simulink model "Assignment2_Simulink"  (R2022b)
settings: Solver=FixedStepAuto  StartTime=0.0  StopTime=20  FixedStep=0.1  RelTol=1e-3
undefined symbols (not defined in the file or in its folder): Ad, Bd, Cd, Dd, k_LQR
libraries: mpclib x6
settings Model: Creator=Alireza  LastModifiedBy=Alireza

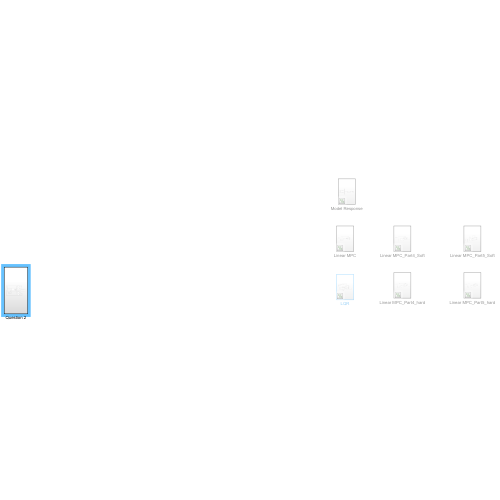
[thumbnail: Simulink's stored preview of the top-level diagram]
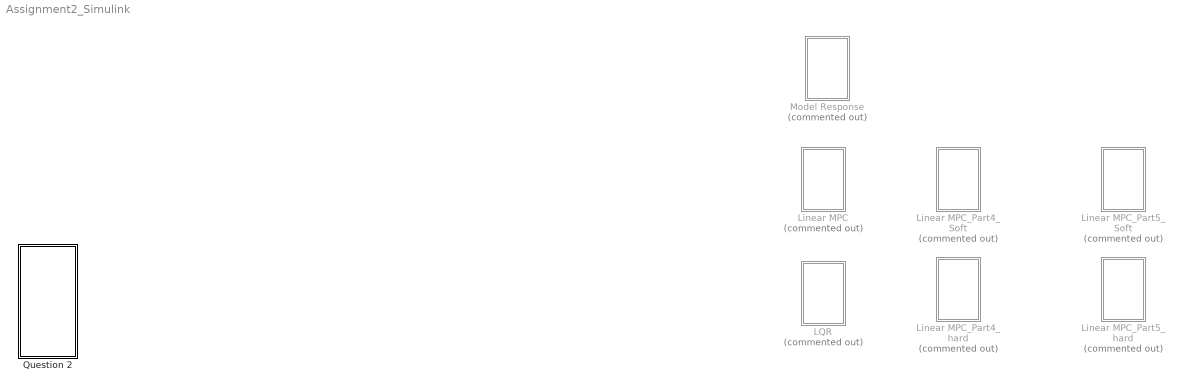
== system Assignment2_Simulink ==
  LQR : Subsystem  Commented=on
  Linear MPC : Subsystem  Commented=on
  Linear MPC_Part4_Soft : Subsystem  Commented=on
  Linear MPC_Part4_hard : Subsystem  Commented=on
  Linear MPC_Part5_Soft : Subsystem  Commented=on
  Linear MPC_Part5_hard : Subsystem  Commented=on
  Model Response : Subsystem  Commented=on
  Question 2 : Subsystem

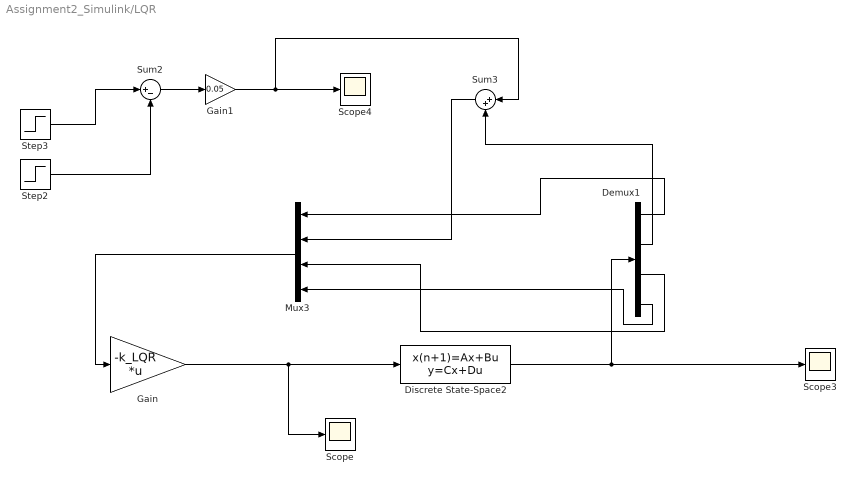
== system Assignment2_Simulink/LQR ==
  Demux1 : Demux
  Discrete State-Space2 : DiscreteStateSpace  A=Ad  B=Bd  C=Cd  D=Dd  InitialCondition=[0,0.1,0,0]  SampleTime=0.1
  Gain : Gain  Gain=-k_LQR  Multiplication=Matrix(K*u)
  Gain1 : Gain  Gain=0.05
  Mux3 : Mux
  Scope : Scope
  Scope3 : Scope
  Scope4 : Scope
  Step2 : Step  Time=5  SampleTime=0
  Step3 : Step  Time=4  SampleTime=0
  Sum2 : Sum  Inputs=|+-
  Sum3 : Sum  Inputs=|++
  wires:
  Demux1/1 -> Mux3/1
  Demux1/3 -> Mux3/3
  Demux1/4 -> Mux3/4
  Sum3/1 -> Mux3/2
  Gain/1 -> Scope/1, Discrete State-Space2/1
  Discrete State-Space2/1 -> Scope3/1, Demux1/1
  Demux1/2 -> Sum3/2
  Step3/1 -> Sum2/1
  Step2/1 -> Sum2/2
  Mux3/1 -> Gain/1
  Sum2/1 -> Gain1/1
  Gain1/1 -> Sum3/1, Scope4/1

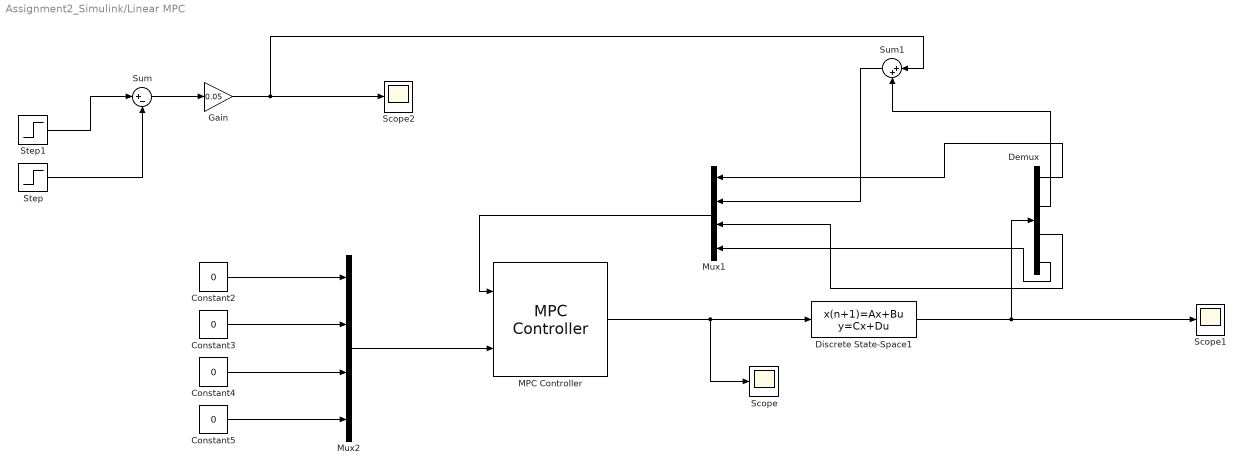
== system Assignment2_Simulink/Linear MPC ==
  Constant{2..5} (4 alike) : Constant  Value=0
  Demux : Demux
  Discrete State-Space1 : DiscreteStateSpace  A=Ad  B=Bd  C=Cd  D=Dd  InitialCondition=[0,0.1,0,0]  SampleTime=0.1
  Gain : Gain  Gain=0.05
  MPC Controller : mpclib/MPC Controller  SCDEnableBlockLinearizationSpecification=on  mpcobj=mpc1  is_multiple=0  enable_value=0  return_u0=off  updateMPCinCallerWorkspace=on  md_inport=off  mv_inport=off  uref_inport=off  return_cost=off  return_mvseq=off  return_qpstatus=off  return_xseq=off  return_state=off  return_ovseq=off  state_inport=off  umin_inport=off  umax_inport=off  ymin_inport=off  ymax_inport=off  cc_inport=off  ywt_inport=off  uwt_inport=off  duwt_inport=off  rhoeps_inport=off  pm_inport=off  MaximumP=10  HorizonChoice=FixedHorizon  n_ts=0.1  n_p=20  n_mv=2  n_md=0  n_ud=0  n_mo=4  n_uo=0  BlockDataType=double  SampleTimeInherited=off  switch_inport=off
  Mux1 : Mux
  Mux2 : Mux
  Scope : Scope
  Scope1 : Scope
  Scope2 : Scope
  Step : Step  Time=5  SampleTime=0
  Step1 : Step  Time=4  SampleTime=0
  Sum : Sum  Inputs=|+-
  Sum1 : Sum  Inputs=|++
  wires:
  Sum1/1 -> Mux1/2
  Step1/1 -> Sum/1
  Discrete State-Space1/1 -> Demux/1, Scope1/1
  Mux2/1 -> MPC Controller/2
  Step/1 -> Sum/2
  Constant3/1 -> Mux2/2
  Mux1/1 -> MPC Controller/1
  Demux/4 -> Mux1/4
  Demux/3 -> Mux1/3
  Constant4/1 -> Mux2/3
  Demux/1 -> Mux1/1
  Constant5/1 -> Mux2/4
  MPC Controller/1 -> Scope/1, Discrete State-Space1/1
  Constant2/1 -> Mux2/1
  Demux/2 -> Sum1/2
  Sum/1 -> Gain/1
  Gain/1 -> Sum1/1, Scope2/1

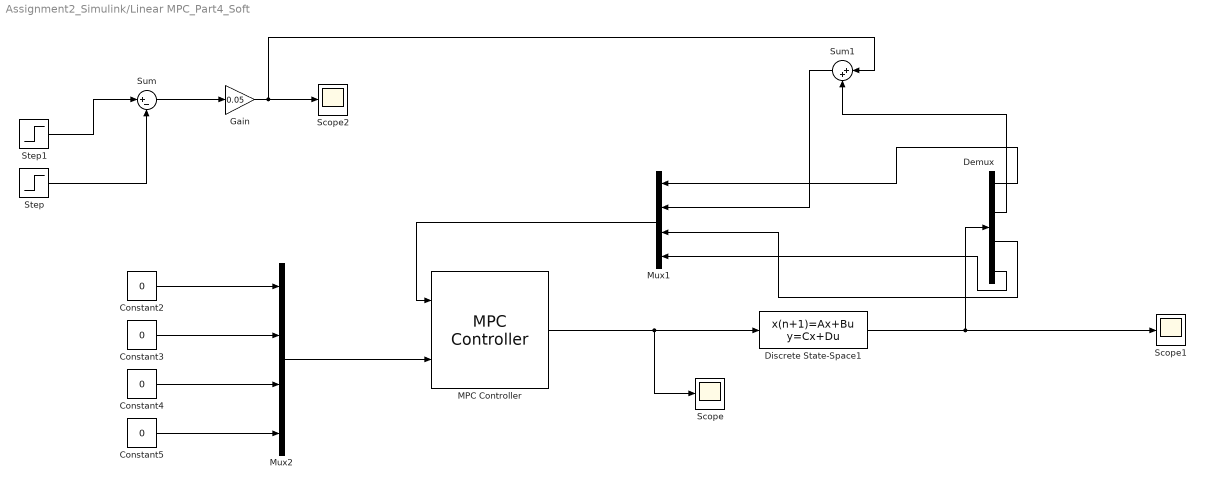
== system Assignment2_Simulink/Linear MPC_Part4_Soft ==
  Constant{2..5} (4 alike) : Constant  Value=0
  Demux : Demux
  Discrete State-Space1 : DiscreteStateSpace  A=Ad  B=Bd  C=Cd  D=Dd  InitialCondition=[0,0.1,0,0]  SampleTime=0.1
  Gain : Gain  Gain=0.05
  MPC Controller : mpclib/MPC Controller  SCDEnableBlockLinearizationSpecification=on  mpcobj=MPC_Part4_Soft  is_multiple=0  enable_value=0  return_u0=off  updateMPCinCallerWorkspace=on  md_inport=off  mv_inport=off  uref_inport=off  return_cost=off  return_mvseq=off  return_qpstatus=off  return_xseq=off  return_state=off  return_ovseq=off  state_inport=off  umin_inport=off  umax_inport=off  ymin_inport=off  ymax_inport=off  cc_inport=off  ywt_inport=off  uwt_inport=off  duwt_inport=off  rhoeps_inport=off  pm_inport=off  MaximumP=10  HorizonChoice=FixedHorizon  n_ts=0.1  n_p=20  n_mv=2  n_md=0  n_ud=0  n_mo=4  n_uo=0  BlockDataType=double  SampleTimeInherited=off  switch_inport=off
  Mux1 : Mux
  Mux2 : Mux
  Scope : Scope
  Scope1 : Scope
  Scope2 : Scope
  Step : Step  Time=5  SampleTime=0
  Step1 : Step  Time=4  SampleTime=0
  Sum : Sum  Inputs=|+-
  Sum1 : Sum  Inputs=|++
  wires:
  Demux/2 -> Sum1/2
  Constant2/1 -> Mux2/1
  MPC Controller/1 -> Discrete State-Space1/1, Scope/1
  Constant5/1 -> Mux2/4
  Demux/1 -> Mux1/1
  Constant4/1 -> Mux2/3
  Demux/3 -> Mux1/3
  Demux/4 -> Mux1/4
  Mux1/1 -> MPC Controller/1
  Constant3/1 -> Mux2/2
  Step/1 -> Sum/2
  Mux2/1 -> MPC Controller/2
  Discrete State-Space1/1 -> Scope1/1, Demux/1
  Step1/1 -> Sum/1
  Sum1/1 -> Mux1/2
  Gain/1 -> Sum1/1, Scope2/1
  Sum/1 -> Gain/1

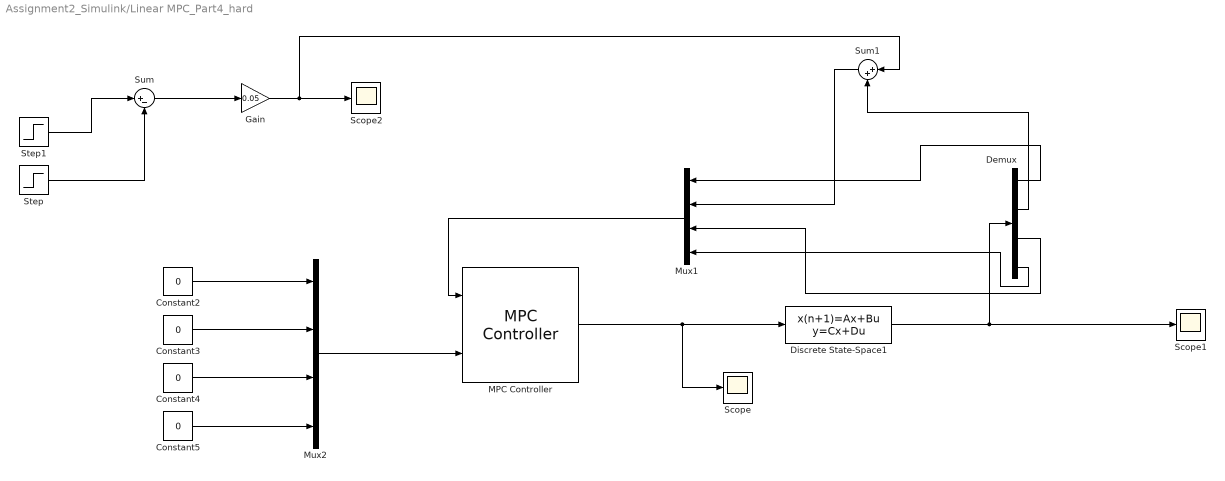
== system Assignment2_Simulink/Linear MPC_Part4_hard ==
  Constant{2..5} (4 alike) : Constant  Value=0
  Demux : Demux
  Discrete State-Space1 : DiscreteStateSpace  A=Ad  B=Bd  C=Cd  D=Dd  InitialCondition=[0,0.1,0,0]  SampleTime=0.1
  Gain : Gain  Gain=0.05
  MPC Controller : mpclib/MPC Controller  SCDEnableBlockLinearizationSpecification=on  mpcobj=MPC_Part4_Hard  is_multiple=0  enable_value=0  return_u0=off  updateMPCinCallerWorkspace=on  md_inport=off  mv_inport=off  uref_inport=off  return_cost=off  return_mvseq=off  return_qpstatus=off  return_xseq=off  return_state=off  return_ovseq=off  state_inport=off  umin_inport=off  umax_inport=off  ymin_inport=off  ymax_inport=off  cc_inport=off  ywt_inport=off  uwt_inport=off  duwt_inport=off  rhoeps_inport=off  pm_inport=off  MaximumP=10  HorizonChoice=FixedHorizon  n_ts=0.1  n_p=20  n_mv=2  n_md=0  n_ud=0  n_mo=4  n_uo=0  BlockDataType=double  SampleTimeInherited=off  switch_inport=off
  Mux1 : Mux
  Mux2 : Mux
  Scope : Scope
  Scope1 : Scope
  Scope2 : Scope
  Step : Step  Time=5  SampleTime=0
  Step1 : Step  Time=4  SampleTime=0
  Sum : Sum  Inputs=|+-
  Sum1 : Sum  Inputs=|++
  wires:
  Sum1/1 -> Mux1/2
  Step1/1 -> Sum/1
  Discrete State-Space1/1 -> Demux/1, Scope1/1
  Mux2/1 -> MPC Controller/2
  Step/1 -> Sum/2
  Constant3/1 -> Mux2/2
  Mux1/1 -> MPC Controller/1
  Demux/4 -> Mux1/4
  Demux/3 -> Mux1/3
  Constant4/1 -> Mux2/3
  Demux/1 -> Mux1/1
  Constant5/1 -> Mux2/4
  MPC Controller/1 -> Scope/1, Discrete State-Space1/1
  Constant2/1 -> Mux2/1
  Demux/2 -> Sum1/2
  Sum/1 -> Gain/1
  Gain/1 -> Sum1/1, Scope2/1

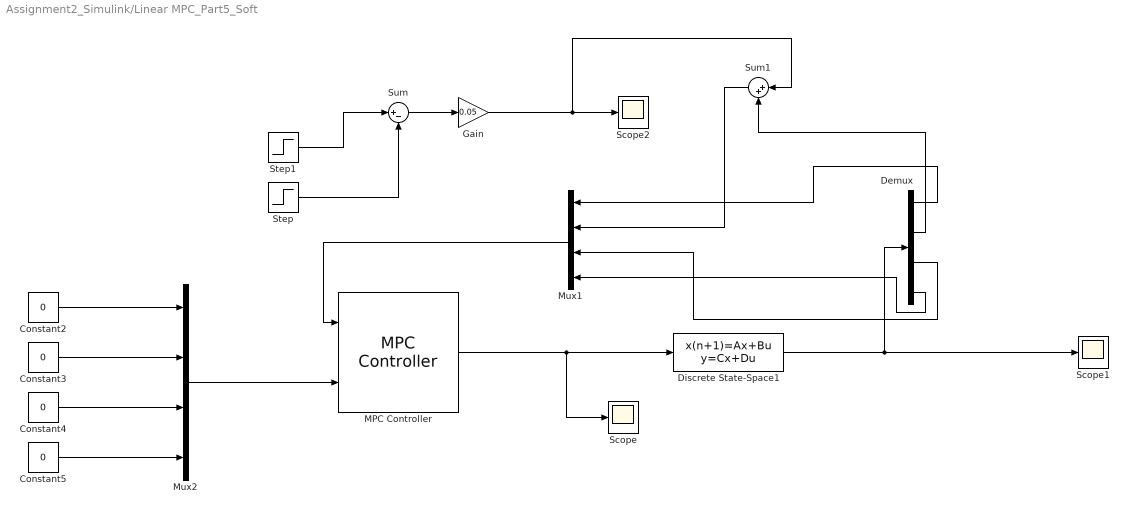
== system Assignment2_Simulink/Linear MPC_Part5_Soft ==
  Constant{2..5} (4 alike) : Constant  Value=0
  Demux : Demux
  Discrete State-Space1 : DiscreteStateSpace  A=Ad  B=Bd  C=Cd  D=Dd  InitialCondition=[0,0.1,0,0]  SampleTime=0.1
  Gain : Gain  Gain=0.05
  MPC Controller : mpclib/MPC Controller  SCDEnableBlockLinearizationSpecification=on  mpcobj=MPC_Part5_Soft  is_multiple=0  enable_value=0  return_u0=off  updateMPCinCallerWorkspace=on  md_inport=off  mv_inport=off  uref_inport=off  return_cost=off  return_mvseq=off  return_qpstatus=off  return_xseq=off  return_state=off  return_ovseq=off  state_inport=off  umin_inport=off  umax_inport=off  ymin_inport=off  ymax_inport=off  cc_inport=off  ywt_inport=off  uwt_inport=off  duwt_inport=off  rhoeps_inport=off  pm_inport=off  MaximumP=10  HorizonChoice=FixedHorizon  n_ts=0.1  n_p=20  n_mv=2  n_md=0  n_ud=0  n_mo=4  n_uo=0  BlockDataType=double  SampleTimeInherited=off  switch_inport=off
  Mux1 : Mux
  Mux2 : Mux
  Scope : Scope
  Scope1 : Scope
  Scope2 : Scope
  Step : Step  Time=5  SampleTime=0
  Step1 : Step  Time=4  SampleTime=0
  Sum : Sum  Inputs=|+-
  Sum1 : Sum  Inputs=|++
  wires:
  Sum1/1 -> Mux1/2
  Step1/1 -> Sum/1
  Discrete State-Space1/1 -> Demux/1, Scope1/1
  Mux2/1 -> MPC Controller/2
  Step/1 -> Sum/2
  Constant3/1 -> Mux2/2
  Mux1/1 -> MPC Controller/1
  Demux/4 -> Mux1/4
  Demux/3 -> Mux1/3
  Constant4/1 -> Mux2/3
  Demux/1 -> Mux1/1
  Constant5/1 -> Mux2/4
  MPC Controller/1 -> Scope/1, Discrete State-Space1/1
  Constant2/1 -> Mux2/1
  Demux/2 -> Sum1/2
  Sum/1 -> Gain/1
  Gain/1 -> Sum1/1, Scope2/1

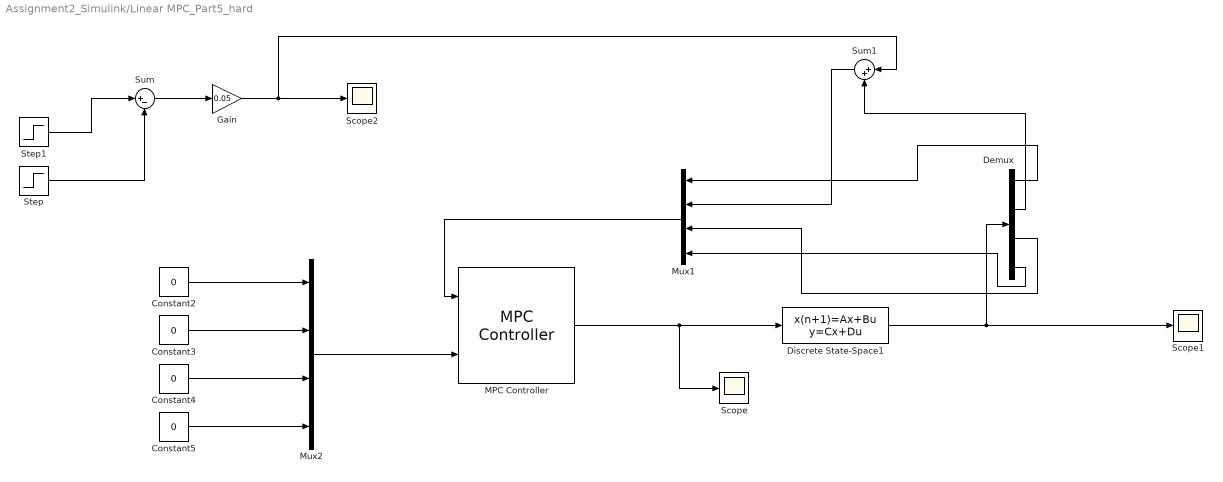
== system Assignment2_Simulink/Linear MPC_Part5_hard ==
  Constant{2..5} (4 alike) : Constant  Value=0
  Demux : Demux
  Discrete State-Space1 : DiscreteStateSpace  A=Ad  B=Bd  C=Cd  D=Dd  InitialCondition=[0,0.1,0,0]  SampleTime=0.1
  Gain : Gain  Gain=0.05
  MPC Controller : mpclib/MPC Controller  SCDEnableBlockLinearizationSpecification=on  mpcobj=MPC_Part5_Hard  is_multiple=0  enable_value=0  return_u0=off  updateMPCinCallerWorkspace=on  md_inport=off  mv_inport=off  uref_inport=off  return_cost=off  return_mvseq=off  return_qpstatus=off  return_xseq=off  return_state=off  return_ovseq=off  state_inport=off  umin_inport=off  umax_inport=off  ymin_inport=off  ymax_inport=off  cc_inport=off  ywt_inport=off  uwt_inport=off  duwt_inport=off  rhoeps_inport=off  pm_inport=off  MaximumP=10  HorizonChoice=FixedHorizon  n_ts=0.1  n_p=20  n_mv=2  n_md=0  n_ud=0  n_mo=4  n_uo=0  BlockDataType=double  SampleTimeInherited=off  switch_inport=off
  Mux1 : Mux
  Mux2 : Mux
  Scope : Scope
  Scope1 : Scope
  Scope2 : Scope
  Step : Step  Time=5  SampleTime=0
  Step1 : Step  Time=4  SampleTime=0
  Sum : Sum  Inputs=|+-
  Sum1 : Sum  Inputs=|++
  wires:
  Demux/2 -> Sum1/2
  Constant2/1 -> Mux2/1
  MPC Controller/1 -> Discrete State-Space1/1, Scope/1
  Constant5/1 -> Mux2/4
  Demux/1 -> Mux1/1
  Constant4/1 -> Mux2/3
  Demux/3 -> Mux1/3
  Demux/4 -> Mux1/4
  Mux1/1 -> MPC Controller/1
  Constant3/1 -> Mux2/2
  Step/1 -> Sum/2
  Mux2/1 -> MPC Controller/2
  Discrete State-Space1/1 -> Scope1/1, Demux/1
  Step1/1 -> Sum/1
  Sum1/1 -> Mux1/2
  Sum/1 -> Gain/1
  Gain/1 -> Sum1/1, Scope2/1

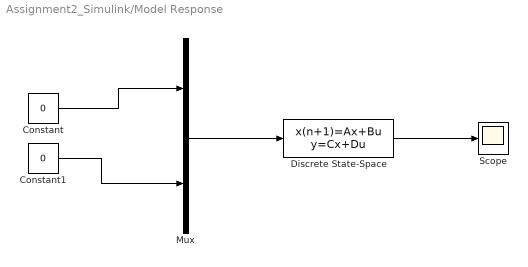
== system Assignment2_Simulink/Model Response ==
  Constant : Constant  Value=0
  Constant1 : Constant  Value=0
  Discrete State-Space : DiscreteStateSpace  A=Ad  B=Bd  C=Cd  D=Dd  InitialCondition=[0,0.1,0,0]  SampleTime=0.1
  Mux : Mux  Inputs=2
  Scope : Scope
  wires:
  Constant/1 -> Mux/1
  Discrete State-Space/1 -> Scope/1
  Constant1/1 -> Mux/2
  Mux/1 -> Discrete State-Space/1

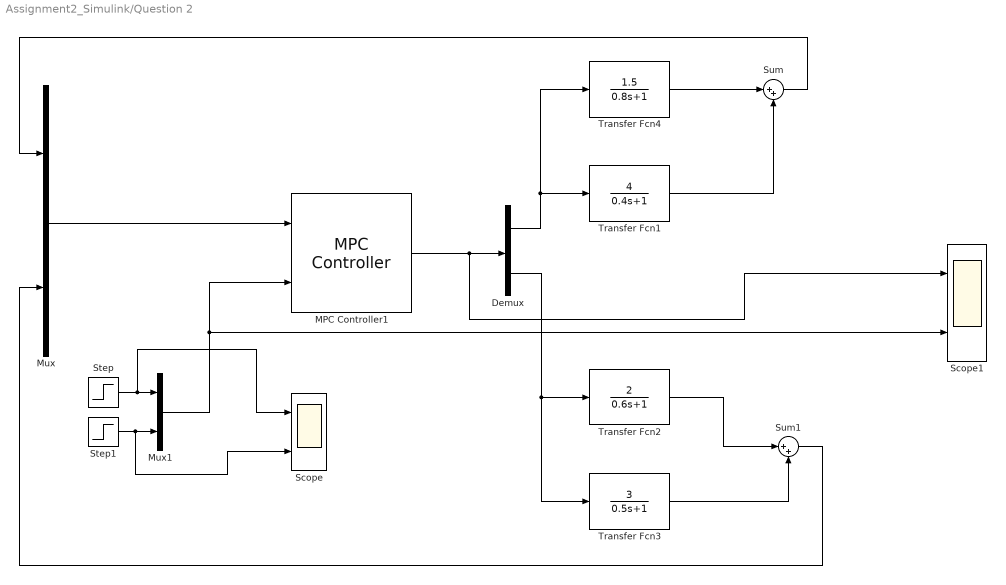
== system Assignment2_Simulink/Question 2 ==
  Demux : Demux  Outputs=2
  MPC Controller1 : mpclib/MPC Controller  SCDEnableBlockLinearizationSpecification=on  mpcobj=mpc1  is_multiple=0  enable_value=0  return_u0=off  updateMPCinCallerWorkspace=on  md_inport=off  mv_inport=off  uref_inport=off  return_cost=off  return_mvseq=off  return_qpstatus=off  return_xseq=off  return_state=off  return_ovseq=off  state_inport=off  umin_inport=off  umax_inport=off  ymin_inport=off  ymax_inport=off  cc_inport=off  ywt_inport=off  uwt_inport=off  duwt_inport=off  rhoeps_inport=off  pm_inport=off  MaximumP=10  HorizonChoice=FixedHorizon  n_ts=0.1  n_p=100  n_mv=2  n_md=0  n_ud=0  n_mo=2  n_uo=0  BlockDataType=double  SampleTimeInherited=off  switch_inport=off
  Mux : Mux  Inputs=2
  Mux1 : Mux  Inputs=2
  Scope : Scope  NumInputPorts=2
  Scope1 : Scope  NumInputPorts=2
  Step : Step  Time=10  Before=-10  After=15  SampleTime=0
  Step1 : Step  Time=5  Before=-20  After=30  SampleTime=0
  Sum : Sum  Inputs=|++
  Sum1 : Sum  Inputs=|++
  Transfer Fcn1 : TransferFcn  Numerator=[4]  Denominator=[0.4 1]
  Transfer Fcn2 : TransferFcn  Numerator=[2]  Denominator=[0.6 1]
  Transfer Fcn3 : TransferFcn  Numerator=[3]  Denominator=[0.5 1]
  Transfer Fcn4 : TransferFcn  Numerator=[1.5]  Denominator=[0.8 1]
  wires:
  Demux/2 -> Transfer Fcn3/1, Transfer Fcn2/1
  Sum1/1 -> Mux/2
  Transfer Fcn1/1 -> Sum/2
  Transfer Fcn3/1 -> Sum1/2
  Sum/1 -> Mux/1
  Transfer Fcn4/1 -> Sum/1
  Mux1/1 -> Scope1/2, MPC Controller1/2
  Transfer Fcn2/1 -> Sum1/1
  Mux/1 -> MPC Controller1/1
  Demux/1 -> Transfer Fcn4/1, Transfer Fcn1/1
  Step/1 -> Scope/1, Mux1/1
  Step1/1 -> Scope/2, Mux1/2
  MPC Controller1/1 -> Scope1/1, Demux/1
